simulink library "MonitoringSystem"  (R2015b)
settings: Solver=VariableStepAuto  StartTime=0.0  StopTime=10.0  RelTol=1e-3
libraries: simulink x1, dspnetwork x1
settings Model: Creator=Ryuu  LastModifiedBy=Ryuu

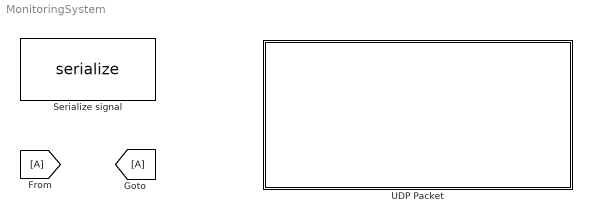
== system MonitoringSystem ==
  Serialize signal : M-S-Function  FunctionName=serialize  Parameters=label, signal_type, min, max  mask(Signal Serializer){label='', signal_type=Type a, min=0, max=0}
      mask prompts: signal_type "Signal Type:"; min "Minimum Safe Value:"; max "Maximum Safe Value:"
      mask help:
      | Define and serialize a signal.
      |
      | Label: The name of the signal.
      | Type: The type of the signal, so units can be added automatically.
      | Minimum Safe Value: The lowest value that is considered safe.
      | Maximum Safe Value: The highes value that is considered safe.
      mask TypeOptions signal_type: Type a | Type b | Type c | Type d | Type e | Type f | Type g | Type h | Type i | Type j | Type k | Type l | Type m | Type n
      mask Display: port_label('input',1,'value')
  UDP Packet : Subsystem

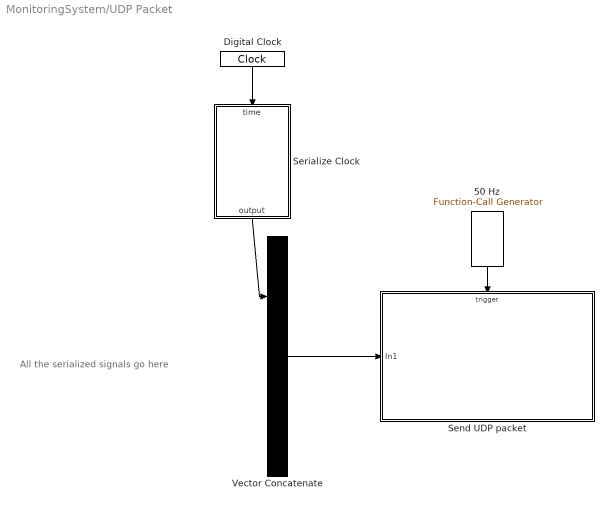
== system MonitoringSystem/UDP Packet ==
  note: All the serialized signals go here
  50 Hz : simulink/Ports & Subsystems/Function-Call Generator  sample_time=0.02  numberOfIterations=1
  Digital Clock : DigitalClock  SampleTime=0.001
  Send UDP packet : Subsystem
  Serialize Clock : MATLAB Function  TreatAsAtomicUnit=on
  Vector Concatenate : Concatenate
  wires:
  50 Hz/1 -> Send UDP packet/Trigger
  Digital Clock/1 -> Serialize Clock/1(time)
  Vector Concatenate/1 -> Send UDP packet/1(In1)
  Serialize Clock/1(output) -> Vector Concatenate/1

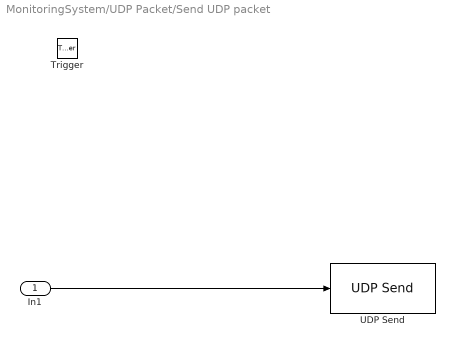
== system MonitoringSystem/UDP Packet/Send UDP packet ==
  In1 : Inport
  Trigger : TriggerPort  TriggerType=function-call  PortDimensions=1
  UDP Send : dspnetwork/UDP Send  remoteURL='127.0.0.1'  remotePort=25000  localURL='0.0.0.0'  localPortSource=Automatically determine  localPort=-1  sampletime=-1  separateLengthPort=0
  wires:
  In1/1 -> UDP Send/1

== matlab function MonitoringSystem/UDP Packet/Serialize Clock ==
  data: time input; output output
function output = time_serialize(time)

time_ser = serialize(time);
output = time_ser;
end


function m = serialize(v)
    % dispatch according to type
    if isnumeric(v) 
        m = serialize_numeric(v);
    elseif ischar(v)
        m = serialize_string(v);
    elseif islogical(v)
        m = serialize_logical(v);
	else
		error('Unsupported data type');
    end
end

% single scalar
function m = serialize_scalar(v)
    % Data type & data
    m = [class2tag(class(v)); typecast(v,'uint8').'];
end

% char arrays
function m = serialize_string(v)
    if size(v,1) == 1
        % horizontal string: Type, Length, and Data
        m = [uint8(0); typecast(uint32(length(v)),'uint8').'; uint8(v(:))];
    elseif sum(size(v)) == 0
        % '': special encoding
        m = uint8(200);
    else
        % general char array: Tag & Number of dimensions, Dimensions, Data
        m = [uint8(132); ndims(v); typecast(uint32(size(v)),'uint8').'; uint8(v(:))];
    end
end

% logical arrays
function m = serialize_logical(v)
    % Tag & Number of dimensions, Dimensions, Data
    m = [uint8(133); ndims(v); typecast(uint32(size(v)),'uint8').'; uint8(v(:))];
end

% non-complex and non-sparse numerical matrix
function m = serialize_numeric_simple(v)
    % Tag & Number of dimensions, Dimensions, Data
    m = [16+class2tag(class(v)); ndims(v); typecast(uint32(size(v)),'uint8').'; typecast(v(:).','uint8').'];
end

% Numeric Matrix: can be real/complex, sparse/full, scalar
function m = serialize_numeric(v)
    if issparse(v)
        % Data Type & Dimensions
        m = [uint8(130); typecast(uint64(size(v,1)), 'uint8').'; typecast(uint64(size(v,2)), 'uint8').']; % vectorize
        % Index vectors
        [i,j,s] = find(v);        
        % Real/Complex
        if isreal(v)
            m = [m; serialize_numeric_simple(i); serialize_numeric_simple(j); 1; serialize_numeric_simple(s)];
        else
            m = [m; serialize_numeric_simple(i); serialize_numeric_simple(j); 0; serialize_numeric_simple(real(s)); serialize_numeric_simple(imag(s))];
        end
    elseif ~isreal(v)
        % Data type & contents
        m = [uint8(131); serialize_numeric_simple(real(v)); serialize_numeric_simple(imag(v))];
    elseif isscalar(v)
        % Scalar
        m = serialize_scalar(v);
    else
        % Simple matrix
        m = serialize_numeric_simple(v);
    end
end

% *container* class to byte
function b = class2tag(cls)
	switch cls
		case 'string'
            b = uint8(0);
		case 'double'
			b = uint8(1);
		case 'single'
			b = uint8(2);
		case 'int8'
			b = uint8(3);
		case 'uint8'
			b = uint8(4);
		case 'int16'
			b = uint8(5);
		case 'uint16'
			b = uint8(6);
		case 'int32'
			b = uint8(7);
		case 'uint32'
			b = uint8(8);
		case 'int64'
			b = uint8(9);
		case 'uint64'
			b = uint8(10);
		otherwise
			error('Unknown class');
    end
end
